simulink model "kp_simulink"  (R2017b)
settings: Solver=VariableStepAuto  StartTime=0.0  StopTime=20  RelTol=1e-3
values from neighbouring files (symbols this model uses):
  A = [-b/J K/J; -K/L R/L]    [distance.m]    (also in kp_script.m = [0 -1/(R*CS); 0 0]; model_params.m; observador_script.m)
  B = [0;1/L]    [distance.m]    (also in kp_script.m = [0 ; -1/(R*CS)]; model_params.m; observador_script.m)
  h = mean(t)/1e6    [get_model.m]    (also in kp_script.m = 0.05; observador_script.m = 0.00527)
  k = acker(A, B, pols)    [kp_script.m]    (also in observador_script.m)
  k1 = kd(1)    [kp_script.m]    (also in observador_script.m = k(1))
  k2 = kd(2)    [kp_script.m]    (also in observador_script.m = k(2))
  kd = acker(Ad, Bd, polsd)    [kp_script.m]    (also in observador_script.m)
  Nu = N(3)    [kp_script.m]    (also in observador_script.m)
  Nx = N(1:2)    [kp_script.m]    (also in observador_script.m)
settings Model: Creator=DNI 53865091  LastModifiedBy=guillem.casado

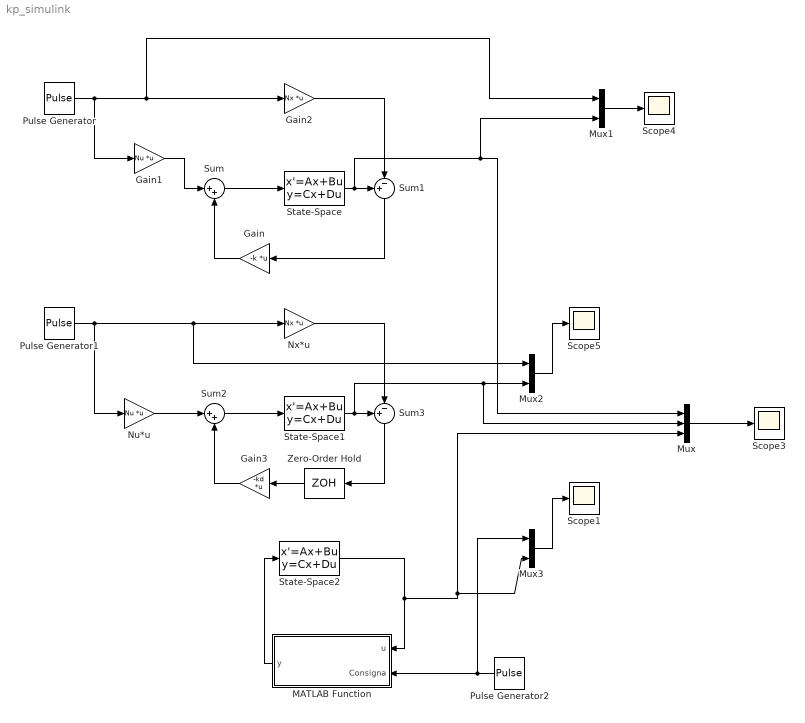
== system kp_simulink ==
  Gain : Gain  Gain=-k  Multiplication=Matrix(K*u)
  Gain1 : Gain  Gain=Nu  Multiplication=Matrix(K*u)
  Gain2 : Gain  Gain=Nx  Multiplication=Matrix(K*u)
  Gain3 : Gain  Gain=-kd  Multiplication=Matrix(K*u)
  MATLAB Function : MATLAB Function  TreatAsAtomicUnit=on
  Mux : Mux  Inputs=3
  Mux1 : Mux  Inputs=2
  Mux2 : Mux  Inputs=2
  Mux3 : Mux  Inputs=2
  Nu*u : Gain  Gain=Nu  Multiplication=Matrix(K*u)
  Nx*u : Gain  Gain=Nx  Multiplication=Matrix(K*u)
  Pulse Generator : DiscretePulseGenerator  PulseType=Time based  Period=5  PulseWidth=50
  Pulse Generator1 : DiscretePulseGenerator  PulseType=Time based  Period=5  PulseWidth=50
  Pulse Generator2 : DiscretePulseGenerator  PulseType=Time based  Period=5  PulseWidth=50
  Scope{1,3..5} (4 alike) : Scope
  State-Space : StateSpace  A=A  B=B  C=eye(2)  D=[0;0]  InitialCondition=[0;1]
  State-Space1 : StateSpace  A=A  B=B  C=eye(2)  D=[0;0]  InitialCondition=[0;1]
  State-Space2 : StateSpace  A=A  B=B  C=eye(2)  D=[0;0]  InitialCondition=[0;1]
  Sum : Sum  Inputs=|++
  Sum1 : Sum  Inputs=+-|
  Sum2 : Sum  Inputs=|++
  Sum3 : Sum  Inputs=+-|
  Zero-Order Hold : ZeroOrderHold  SampleTime=h
  wires:
  Gain/1 -> Sum/2
  Sum/1 -> State-Space/1
  State-Space/1 -> Mux1/2, Mux/1, Sum1/1
  Sum1/1 -> Gain/1
  Pulse Generator/1 -> Gain1/1, Mux1/1, Gain2/1
  Gain1/1 -> Sum/1
  Gain2/1 -> Sum1/2
  Nx*u/1 -> Sum3/2
  Nu*u/1 -> Sum2/1
  Pulse Generator1/1 -> Mux2/1, Nx*u/1, Nu*u/1
  Sum3/1 -> Zero-Order Hold/1
  State-Space1/1 -> Sum3/1, Mux2/2, Mux/2
  Sum2/1 -> State-Space1/1
  Gain3/1 -> Sum2/2
  Zero-Order Hold/1 -> Gain3/1
  MATLAB Function/1(y) -> State-Space2/1
  State-Space2/1 -> Mux3/2, Mux/3, MATLAB Function/1(u)
  Mux/1 -> Scope3/1
  Mux1/1 -> Scope4/1
  Mux2/1 -> Scope5/1
  Mux3/1 -> Scope1/1
  Pulse Generator2/1 -> Mux3/1, MATLAB Function/2(Consigna)

== matlab function kp_simulink/MATLAB Function ==
  settings: updateMethod=DISCRETE  sampleTime=h
  data: u input size=2; y output size=1; k1 parameter; k2 parameter; Consigna input size=1; Nx parameter size=2; Nu parameter size=1
function y = fcn(u,k1, k2, Consigna, Nx, Nu)
ConsNx1 = Nx(1) * Consigna;
ConsNx2 = Nx(2) * Consigna;
ConsNu = Nu * Consigna;
uNx1 = u(1)-ConsNx1;
uNx2 = u(2)-ConsNx2;
uNxK= uNx1*-k1 + uNx2*-k2;
y = uNxK+ConsNu;
